simulink model "lab_6_sl"  (R2021b)
settings: Solver=ode4  StartTime=0.0  StopTime=50.0  FixedStep=2^-5  RelTol=1e-3
settings Model: Creator=JaSzw  LastModifiedBy=JaSzw

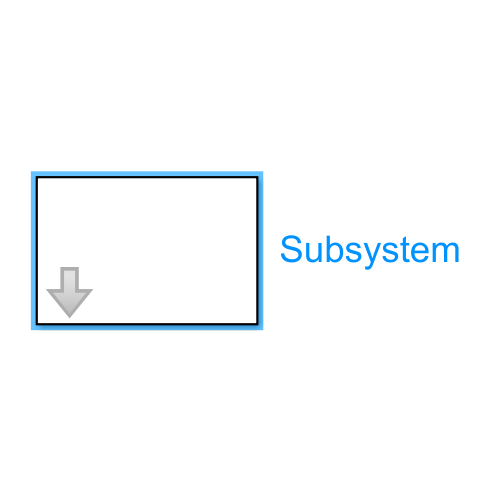
[thumbnail: Simulink's stored preview of the top-level diagram]
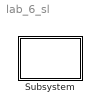
== system lab_6_sl ==
  Subsystem : Subsystem  mask{g=9.81, m1=1, m2=3, M=1, R=0.001}
      mask prompts: g "przyspieszenie ziemskie"; m1 "masa wahadła"; m2 "masa ciężarka"; M "masa bloczków"; R "promień bloczków"

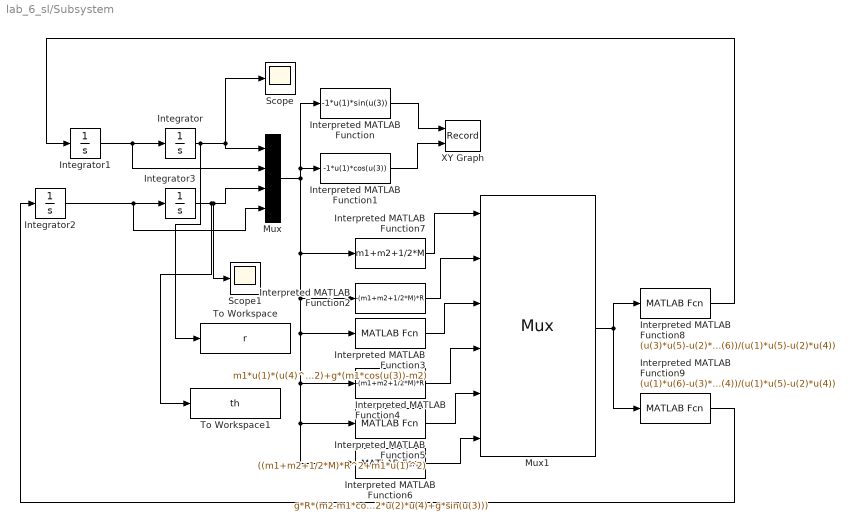
== system lab_6_sl/Subsystem ==
  Integrator : Integrator  InitialCondition=1
  Integrator1 : Integrator
  Integrator2 : Integrator
  Integrator3 : Integrator  InitialCondition=90*pi/180
  Interpreted MATLAB Function : MATLABFcn  MATLABFcn=-1*u(1)*sin(u(3))  OutputDimensions=1
  Interpreted MATLAB Function1 : MATLABFcn  MATLABFcn=-1*u(1)*cos(u(3))  OutputDimensions=1
  Interpreted MATLAB Function2 : MATLABFcn  MATLABFcn=-(m1+m2+1/2*M)*R  OutputDimensions=1
  Interpreted MATLAB Function3 : MATLABFcn  MATLABFcn=m1*u(1)*(u(4)^2)+g*(m1*cos(u(3))-m2)  OutputDimensions=1
  Interpreted MATLAB Function4 : MATLABFcn  MATLABFcn=-(m1+m2+1/2*M)*R  OutputDimensions=1
  Interpreted MATLAB Function5 : MATLABFcn  MATLABFcn=((m1+m2+1/2*M)*R^2+m1*u(1)^2)  OutputDimensions=1
  Interpreted MATLAB Function6 : MATLABFcn  MATLABFcn=g*R*(m2-m1*cos(u(3)))-m1*u(1)*(2*u(2)*u(4)+g*sin(u(3)))  OutputDimensions=1
  Interpreted MATLAB Function7 : MATLABFcn  MATLABFcn=m1+m2+1/2*M  OutputDimensions=1
  Interpreted MATLAB Function8 : MATLABFcn  MATLABFcn=(u(3)*u(5)-u(2)*u(6))/(u(1)*u(5)-u(2)*u(4))  OutputDimensions=1
  Interpreted MATLAB Function9 : MATLABFcn  MATLABFcn=(u(1)*u(6)-u(3)*u(4))/(u(1)*u(5)-u(2)*u(4))  OutputDimensions=1
  Mux : Mux
  Mux1 : Mux  Inputs=6
  Scope : Scope
  Scope1 : Scope
  To Workspace : ToWorkspace  VariableName=r  SampleTime=-1
  To Workspace1 : ToWorkspace  VariableName=th  SampleTime=-1
  XY Graph : Record  FileSettingsInternal="{\"entries\":[{\"content\":{\"excelSettings\":{\"content\":{},\"type\":\"Streamout.ExcelSettings\"}},\"type\":\"Streamout.FileSettingStorage\",\"uuid\":\"83c0cad9-f886-4eea-8c48-5fe786f18ded\"}],\"packageUris\":[\"http://schema.mathworks.com/mf0/streamout_blocks/R2020a\"],\"version\":\"1.0\"}"  Layout=[1 1]  SignalsInternal="{\"entries\":[{\"content\":{\"signals\":[{\"content\":{\"blockPath\":[\"lab_6_sl/Subsystem/XY Graph\"],\"channel\":[],\"dimensions\":[1],\"domain\":\"lab_6_sl/Subsystem/XY Graph\",\"lineColor\":\"#a2142f\",\"plots\":[1],\"port\":1,\"sid\":[\"\"],\"signalID\":181,\"signalName\":\"Interpreted MATLAB\\nFunction\"},\"type\":\"RecordBlkView.Signal\",\"uuid\":\"f7aa5f15-6589-4932-8f15-c99361aa117f\"},{\"content\":{\"blockPath\":[\"lab_6_sl/Subsystem/XY Graph\"],\"channel\":[],\"dimensions\":[1],\"domain\":\"lab_6_sl/Subsystem/XY Graph\",\"lineColor\":\"#139fff\",\"plots\":[1],\"port\":2,\"sid\":[\"\"],\"signalID\":185,\"signalName\":\"Interpreted MATLAB\\nFunction1\"},\"type\":\"RecordBlkView.Signal\",\"uuid\":\"e9e42b44-2ab8-48ad-ad5b-02b4454b57a2\"}]},\"type\":\"RecordBlkView.InputSignals\",\"uuid\":\"ab400e71-1858-4250-85c7-147b54337b82\"}],\"packageUris\":[\"http://schema.mathworks.com/mf0/streamout_blocks/R2020a\"],\"version\":\"1.0\"}"  VisualizationBindings="{\"xyplotplugin\":{\"info\":[{\"series\":[{\"bindingParametersList\":[{\"parameter\":\"X-Axis\",\"signalID\":181,\"signalName\":\"Interpreted MATLAB\\nFunction\"},{\"parameter\":\"Y-Axis\",\"signalID\":185,\"signalName\":\"Interpreted MATLAB\\nFunction1\"}],\"seriesID\":24817}],\"subplotID\":1}]}}"  CompatibilityTag=XY
  wires:
  Interpreted MATLAB Function9/1 -> Integrator2/1
  Mux/1 -> Interpreted MATLAB Function6/1, Interpreted MATLAB Function5/1, Interpreted MATLAB Function4/1, Interpreted MATLAB Function3/1, Interpreted MATLAB Function2/1, Interpreted MATLAB Function7/1, Interpreted MATLAB Function/1, Interpreted MATLAB Function1/1
  Integrator3/1 -> To Workspace1/1, Mux/3, Scope1/1
  Mux1/1 -> Interpreted MATLAB Function9/1, Interpreted MATLAB Function8/1
  Interpreted MATLAB Function3/1 -> Mux1/3
  Interpreted MATLAB Function/1 -> XY Graph/1
  Integrator2/1 -> Integrator3/1, Mux/4
  Integrator/1 -> To Workspace/1, Scope/1, Mux/1
  Interpreted MATLAB Function8/1 -> Integrator1/1
  Interpreted MATLAB Function7/1 -> Mux1/1
  Interpreted MATLAB Function5/1 -> Mux1/5
  Interpreted MATLAB Function6/1 -> Mux1/6
  Interpreted MATLAB Function1/1 -> XY Graph/2
  Interpreted MATLAB Function2/1 -> Mux1/2
  Integrator1/1 -> Mux/2, Integrator/1
  Interpreted MATLAB Function4/1 -> Mux1/4
